simulink model "sm_import_stewart_platform"  (R2021b)
settings: Solver=ode45  StartTime=0.0  StopTime=10.0  RelTol=1e-3  EnableMultiTasking=on
model workspace (MATLAB code in the model file):
  | % The six origin vectors correspond to the six legs of the Stewart platform
  | stewart_pos_base = [0.0962 0 -0.0336; 0.0772 0 -0.0665;-0.0742 0 -0.0599;...
  |     -0.0962 0 -0.0336; -0.0190 0 0.1001;0.019 0 0.1001];
  | 
  | % Corresponding body points on the top plate
  | stewart_body_pts = [0.0607 0 0.0203; 0.0128 0 -0.0628; -0.0145 0 -0.0669; ...
  |     -0.0652 0 0.0208; -0.0507 0 0.046; 0.0507 0 0.046]';
  | 
  | % Leg length
  | leg_length = 0.19*ones(1,6);
undefined symbols (not defined in the file): X, Y, Z
libraries: sm_lib x1374, nesl_utility x19
(part 28 of 28)

== system sm_import_stewart_platform/Stewart Platform/Imported Stewart Platform/BaseRingAssembly_1_RIGID/SwivelBearing6_1_RIGID/swivelbearingbase_1_RIGID/MPB_C345MB_1_RIGID ==
  ReferenceFrame : sm_lib/Frames and Transforms/Reference Frame
  Solid : sm_lib/Body Elements/File Solid  ExtGeomFileName=MPB_C345MB_Default_sldprt.STL  UnitType=Custom  ExtGeomFileUnits=cm  StepReaderType=HEX  ExportConvexHullGeometry=off  InertiaType=Custom  Mass=0.0062849071527897923  MassUnits=kg  CenterOfMass=[-0.0046795799911488294 0.00015178157130363607 0]  CenterOfMassUnits=cm  MomentsOfInertia=[0.0022913911278941504 0.0012611416115453757 0.0012599661343779603]  MomentsOfInertiaUnits=kg*cm^2  ProductsOfInertia=[0 -8.795786235852507e-09 -4.4951153027101913e-09]  ProductsOfInertiaUnits=kg*cm^2  BasedOnType=Density  Density=1000  DensityUnits=kg/(m^3)  DoExposeReferenceFrame=on  SerializedFrames=<Frames/>  GraphicType=FromGeometry  MarkerShape=Sphere  MarkerSize=10  MarkerSizeUnits=m  GraphicVisPropType=SimpleVisualProperties  GraphicDiffuseColor=[0.72282352941176464 0.72282352941176464 0.72282352941176464]  GraphicSpecularColor=[0.5 0.5 0.5 1.0]  GraphicAmbientColor=[0.15 0.15 0.15 1.0]  GraphicEmissiveColor=[0.0 0.0 0.0 1.0]  GraphicShininess=75  GraphicOpacity=1
  F : PMIOPort  Side=Left
  connections:
  ReferenceFrame/RConn1 -- Solid/RConn1 -- F/RConn1

== system sm_import_stewart_platform/Stewart Platform/Imported Stewart Platform/BaseRingAssembly_1_RIGID/SwivelBearing6_1_RIGID/swivelbearingbase_1_RIGID/MPB_C345MB_2_RIGID ==
  ReferenceFrame : sm_lib/Frames and Transforms/Reference Frame
  Solid : sm_lib/Body Elements/File Solid  ExtGeomFileName=MPB_C345MB_Default_sldprt.STL  UnitType=Custom  ExtGeomFileUnits=cm  StepReaderType=HEX  ExportConvexHullGeometry=off  InertiaType=Custom  Mass=0.0062849071527897923  MassUnits=kg  CenterOfMass=[-0.0046795799911488294 0.00015178157130363607 0]  CenterOfMassUnits=cm  MomentsOfInertia=[0.0022913911278941504 0.0012611416115453757 0.0012599661343779603]  MomentsOfInertiaUnits=kg*cm^2  ProductsOfInertia=[0 -8.795786235852507e-09 -4.4951153027101913e-09]  ProductsOfInertiaUnits=kg*cm^2  BasedOnType=Density  Density=1000  DensityUnits=kg/(m^3)  DoExposeReferenceFrame=on  SerializedFrames=<Frames/>  GraphicType=FromGeometry  MarkerShape=Sphere  MarkerSize=10  MarkerSizeUnits=m  GraphicVisPropType=SimpleVisualProperties  GraphicDiffuseColor=[0.72282352941176464 0.72282352941176464 0.72282352941176464]  GraphicSpecularColor=[0.5 0.5 0.5 1.0]  GraphicAmbientColor=[0.15 0.15 0.15 1.0]  GraphicEmissiveColor=[0.0 0.0 0.0 1.0]  GraphicShininess=75  GraphicOpacity=1
  F : PMIOPort  Side=Left
  connections:
  ReferenceFrame/RConn1 -- Solid/RConn1 -- F/RConn1

== system sm_import_stewart_platform/Stewart Platform/Imported Stewart Platform/BaseRingAssembly_1_RIGID/SwivelBearing6_1_RIGID/swivelbearingshaft_1_RIGID/Hex_Nut_M5_1_RIGID ==
  ReferenceFrame : sm_lib/Frames and Transforms/Reference Frame
  Solid : sm_lib/Body Elements/File Solid  ExtGeomFileName=Hex_Nut_M5_Default_sldprt.STL  UnitType=Custom  ExtGeomFileUnits=cm  StepReaderType=HEX  ExportConvexHullGeometry=off  InertiaType=Custom  Mass=0.0014621210054577064  MassUnits=kg  CenterOfMass=[0.23500000003652866 8.4057718888777272e-13 -1.6260373351668095e-12]  CenterOfMassUnits=cm  MomentsOfInertia=[0.0001588164272622833 0.00010395888711664299 0.0001039598591326645]  MomentsOfInertiaUnits=kg*cm^2  ProductsOfInertia=[1.1387721654918686e-10 2.0700174573802443e-10 0]  ProductsOfInertiaUnits=kg*cm^2  BasedOnType=Density  Density=1000  DensityUnits=kg/(m^3)  DoExposeReferenceFrame=on  SerializedFrames=<Frames/>  GraphicType=FromGeometry  MarkerShape=Sphere  MarkerSize=10  MarkerSizeUnits=m  GraphicVisPropType=SimpleVisualProperties  GraphicDiffuseColor=[0.77647058823529413 0.75686274509803919 0.73725490196078436]  GraphicSpecularColor=[0.5 0.5 0.5 1.0]  GraphicAmbientColor=[0.15 0.15 0.15 1.0]  GraphicEmissiveColor=[0.0 0.0 0.0 1.0]  GraphicShininess=75  GraphicOpacity=1
  F : PMIOPort  Side=Left
  connections:
  ReferenceFrame/RConn1 -- Solid/RConn1 -- F/RConn1

== system sm_import_stewart_platform/Stewart Platform/Imported Stewart Platform/BaseRingAssembly_1_RIGID/SwivelBearing6_1_RIGID/swivelbearingshaft_1_RIGID/Threaded_Shaft_1_RIGID ==
  ReferenceFrame : sm_lib/Frames and Transforms/Reference Frame
  Solid : sm_lib/Body Elements/File Solid  ExtGeomFileName=Threaded_Shaft_Default_sldprt.STL  UnitType=Custom  ExtGeomFileUnits=cm  StepReaderType=HEX  ExportConvexHullGeometry=off  InertiaType=Custom  Mass=0.0067286771531606558  MassUnits=kg  CenterOfMass=[0 -1.6645365513234152e-08 2.2496640173633495]  CenterOfMassUnits=cm  MomentsOfInertia=[0.011498510043092661 0.011501318043092663 0.00020671437691650223]  MomentsOfInertiaUnits=kg*cm^2  ProductsOfInertia=[1.3542537359420902e-10 0 0]  ProductsOfInertiaUnits=kg*cm^2  BasedOnType=Density  Density=1000  DensityUnits=kg/(m^3)  DoExposeReferenceFrame=on  SerializedFrames=<Frames/>  GraphicType=FromGeometry  MarkerShape=Sphere  MarkerSize=10  MarkerSizeUnits=m  GraphicVisPropType=SimpleVisualProperties  GraphicDiffuseColor=[0.77647058823529413 0.75686274509803919 0.73725490196078436]  GraphicSpecularColor=[0.5 0.5 0.5 1.0]  GraphicAmbientColor=[0.15 0.15 0.15 1.0]  GraphicEmissiveColor=[0.0 0.0 0.0 1.0]  GraphicShininess=75  GraphicOpacity=1
  F : PMIOPort  Side=Left
  connections:
  ReferenceFrame/RConn1 -- Solid/RConn1 -- F/RConn1

== system sm_import_stewart_platform/Stewart Platform/Imported Stewart Platform/BaseRingAssembly_1_RIGID/SwivelBearing6_1_RIGID/swivelbearingshaft_1_RIGID/Yoke_1_RIGID ==
  ReferenceFrame : sm_lib/Frames and Transforms/Reference Frame
  Solid : sm_lib/Body Elements/File Solid  ExtGeomFileName=Yoke_Default_sldprt.STL  UnitType=Custom  ExtGeomFileUnits=m  StepReaderType=HEX  ExportConvexHullGeometry=off  InertiaType=Custom  Mass=0.0085668068985893069  MassUnits=kg  CenterOfMass=[3.3036113322449594e-09 4.5392080360257641e-09 0.013809135161090778]  CenterOfMassUnits=m  MomentsOfInertia=[3.6198630707133227e-07 3.7260728672028368e-07 1.1777278033424778e-07]  MomentsOfInertiaUnits=kg*m^2  ProductsOfInertia=[1.5891854780888145e-13 3.9281797530062808e-13 -1.9646780999777998e-13]  ProductsOfInertiaUnits=kg*m^2  BasedOnType=Density  Density=1000  DensityUnits=kg/(m^3)  DoExposeReferenceFrame=on  SerializedFrames=<Frames/>  GraphicType=FromGeometry  MarkerShape=Sphere  MarkerSize=10  MarkerSizeUnits=m  GraphicVisPropType=SimpleVisualProperties  GraphicDiffuseColor=[0.77647058823529413 0.75686274509803919 0.73725490196078436]  GraphicSpecularColor=[0.5 0.5 0.5 1.0]  GraphicAmbientColor=[0.15 0.15 0.15 1.0]  GraphicEmissiveColor=[0.0 0.0 0.0 1.0]  GraphicShininess=75  GraphicOpacity=1
  F : PMIOPort  Side=Left
  connections:
  ReferenceFrame/RConn1 -- Solid/RConn1 -- F/RConn1
